simulink model "rtwdemo_whileeml"  (Simulink 7.1)
settings: Solver=FixedStepDiscrete  StartTime=0.0  StopTime=10.0  FixedStep=.01  RelTol=1e-3
settings Model: Creator=ajayaram  LastModifiedBy=ajayaram
settings OptimizationCC: InlineParams=on  OptimizeModelRefInitCode=on  LifeSpan=1
settings DebuggingCC: SaveWithParameterizedLinksMsg=none
settings RTWCC: SystemTargetFile=ert.tlc  GenCodeOnly=on  GenerateMakefile=off  TemplateMakefile=ert_default_tmf  Description=Real-Time Workshop Embedded Coder (no auto configuration)  GenerateReport=on  ProcessScript=ert_make_rtw_hook  IncludeHyperlinkInReport=on  LaunchReport=on
settings CodeAppCC: GenerateComments=off  IgnoreCustomStorageClasses=off  SimulinkBlockComments=off
settings ERTTargetCC: TargetFcnLib=ansi_tfl_tmw.mat  GenerateSampleERTMain=on  IncludeMdlTerminateFcn=off  SupportComplex=off  InlinedParameterPlacement=NonHierarchical  ERTCustomFileTemplate=example_file_process.tlc

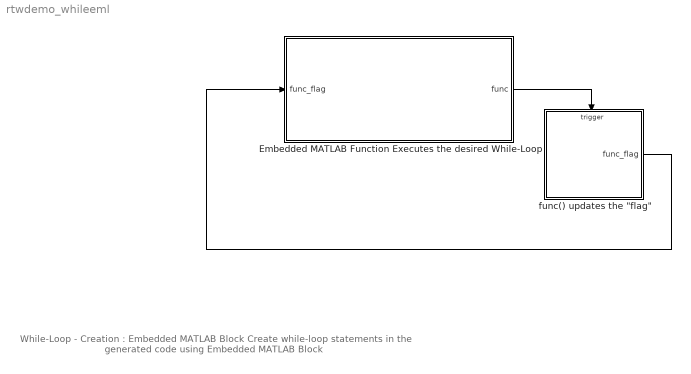
== system rtwdemo_whileeml ==
  note: While-Loop - Creation : Embedded MATLAB Block
      | Create while-loop statements in the
      | generated code using Embedded MATLAB Block
  Embedded MATLAB Function Executes the desired While-Loop : Stateflow chart
  "func() updates the \"flag\"" : Subsystem  RTWFcnName=func
      settings: RTWSystemCode=Function  RTWFcnNameOpts=User specified  RTWFileNameOpts=Use function name
  wires:
  "func() updates the \"flag\""/1(func_flag) -> Embedded MATLAB Function Executes the desired While-Loop/1(func_flag)
  Embedded MATLAB Function Executes the desired While-Loop/1(func) -> "func() updates the \"flag\""/Trigger

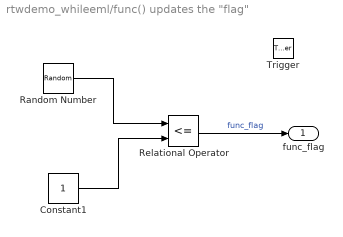
== system rtwdemo_whileeml/func() updates the "flag" ==
  Trigger : TriggerPort  TriggerType=function-call
  Constant1 : Constant  OutDataTypeMode=double  OutDataType=sfix(16)  OutScaling=2^0  OutDataTypeStr=double
  Random Number : RandomNumber
  Relational Operator : RelationalOperator  Operator=<=  LogicOutDataTypeMode=boolean  OutDataTypeStr=boolean
  func_flag : Outport  OutDataType=sfix(16)  OutScaling=2^0
  wires:
  Random Number/1 -> Relational Operator/1
  Constant1/1 -> Relational Operator/2
  Relational Operator/1 -> func_flag/1  "func_flag"

== matlab function Embedded MATLAB Function Executes the desired While-Loop ==
  data: func_flag input double
  events: func output FUNCTION_CALL_EVENT
function fcn(func_flag)

flag = true; num_iter = 1;

while(flag && (num_iter<=100))
    func;
    flag = func_flag;
    num_iter = num_iter + 1;
end
